simulink model "Controller"  (R2021a)
settings: Solver=FixedStepDiscrete  StartTime=0.0  StopTime=10.0  FixedStep=0.005  RelTol=1e-3
settings Model: Creator=ZJO9FE  LastModifiedBy=ZJO9FE
settings DataIOCC: SaveFormat=StructureWithTime
settings OptimizationCC: DefaultParameterBehavior=Inlined  EnhancedBackFolding=on  PassReuseOutputArgsAs=Individual arguments  ZeroExternalMemoryAtStartup=off  ZeroInternalMemoryAtStartup=off  OptimizeBlockOrder=speed  DifferentSizesBufferReuse=on  OptimizationCustomize=off  EfficientTunableParamExpr=on
settings DebuggingCC: ParameterTunabilityLossMsg=error
settings SFSimCC: MATLABDynamicMemAlloc=off
settings RTWCC: Description=AUTOSAR  SystemTargetFile=autosar.tlc  GenCodeOnly=on  TemplateMakefile=ert_default_tmf  GenerateReport=on  LaunchReport=on
settings CodeAppCC: ForceParamTrailComments=on  IgnoreCustomStorageClasses=off  OperatorAnnotations=on  SimulinkDataObjDesc=on  SFDataObjDesc=on  InsertBlockDesc=on
settings STFCustomTargetCC: TargetLangStandard=C99 (ISO)  MultiwordLength=256  ParMdlRefBuildCompliant=on  CompOptLevelCompliant=on  IncludeMdlTerminateFcn=off  CombineOutputUpdateFcns=on  SuppressErrorStatus=on  ERTCustomFileBanners=on  SupportNonFinite=off  SupportComplex=off  SupportContinuousTime=off  SupportNonInlinedSFcns=off  RemoveResetFunc=on  MATLABClassNameForMDSCustomization=Simulink.SoftwareTarget.ERTCustomization  AutosarCompliant=on  GRTInterface=off  LookupTableObjectStructAxisOrder=2,1,3,4,...  LUTObjectStructOrderEvenSpacing=Size,Table,Breakpoints  SystemTargetFile=autosar.tlc
settings ERTTargetCC: TargetLangStandard=C99 (ISO)  ConcurrentExecutionCompliant=off  IncludeMdlTerminateFcn=off  SuppressErrorStatus=on  SupportNonFinite=off  SupportComplex=off  ModelStepFunctionPrototypeControlCompliant=off  CPPClassGenCompliant=off  AutosarCompliant=on  LookupTableObjectStructAxisOrder=2,1,3,4,...  LUTObjectStructOrderEvenSpacing=Size,Table,Breakpoints  InlinedParameterPlacement=NonHierarchical  ERTCustomFileTemplate=example_file_process.tlc

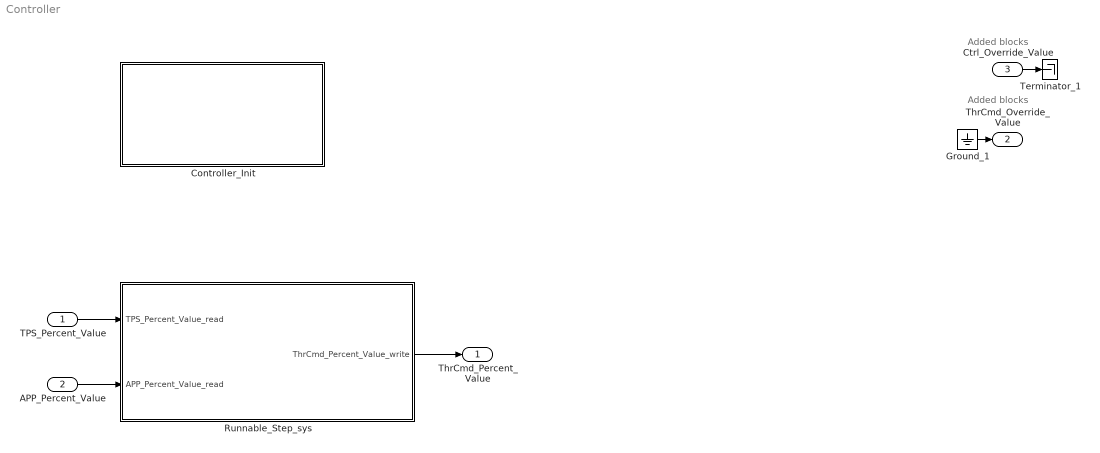
== system Controller ==
  note: Added blocks
  note: Added blocks
  TPS_Percent_Value : Inport  OutDataTypeStr=single  PortDimensions=1
  APP_Percent_Value : Inport  Port=2  OutDataTypeStr=single  PortDimensions=1
  Ctrl_Override_Value : Inport  Port=3  OutDataTypeStr=single  PortDimensions=1
  Controller_Init : Subsystem
  Ground_1 : Ground
  Runnable_Step_sys : Subsystem  TreatAsAtomicUnit=on  SystemSampleTime=0.005
  Terminator_1 : Terminator
  ThrCmd_Percent_Value : Outport  OutDataTypeStr=single  PortDimensions=1
  ThrCmd_Override_Value : Outport  Port=2  OutDataTypeStr=single  PortDimensions=1  SampleTime=0.005
  wires:
  TPS_Percent_Value/1 -> Runnable_Step_sys/1(TPS_Percent_Value_read)
  APP_Percent_Value/1 -> Runnable_Step_sys/2(APP_Percent_Value_read)
  Runnable_Step_sys/1(ThrCmd_Percent_Value_write) -> ThrCmd_Percent_Value/1
  Ctrl_Override_Value/1 -> Terminator_1/1
  Ground_1/1 -> ThrCmd_Override_Value/1

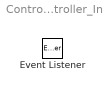
== system Controller/Controller_Init ==
  Event Listener : EventListener  EventName=reset

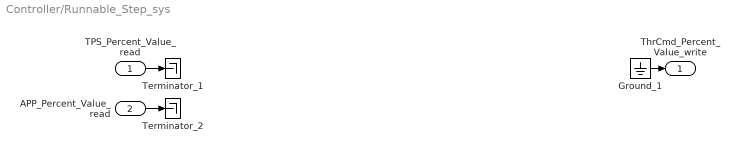
== system Controller/Runnable_Step_sys ==
  TPS_Percent_Value_read : Inport
  APP_Percent_Value_read : Inport  Port=2
  Ground_1 : Ground
  Terminator_1 : Terminator
  Terminator_2 : Terminator
  ThrCmd_Percent_Value_write : Outport
  wires:
  TPS_Percent_Value_read/1 -> Terminator_1/1
  APP_Percent_Value_read/1 -> Terminator_2/1
  Ground_1/1 -> ThrCmd_Percent_Value_write/1
